simulink model "EspacioEstado"  (R2017b)
settings: Solver=VariableStepAuto  StartTime=0.0  StopTime=0.5  MaxStep=1e-4  RelTol=1e-3
values from neighbouring files (symbols this model uses):
  A = pi()*((D/2)^2)    [MODELOHIDRO.m]    (also in MODELOHIDROV10.m; MODELOHIDROV2.m; MODELOHIDROV3.m; MODELOHIDROV4.m)
  B = 0    [MODELOHIDRO.m]    (also in MODELOHIDROV10.m; MODELOHIDROV2.m; MODELOHIDROV3.m; MODELOHIDROV4.m)
  C = [1 0;0 1]    [PruebaDCDC.m]    (also in stateStadeInv.m = [0 0 0 1 0 0;0 0 0 0 1 0;0 0 0 0 0 1])
  Ccc = 2.5e-3    (= 0.0025)    [MODELOHIDROV4.m]    (also in MODELOHIDROV7.m = 8.33e-05; MODELOHIDROV8.m = 8.33e-05; PruebaDCDC.m = 8.33e-05)
  D = 1    [MODELOHIDRO.m]    (also in MODELOHIDROV10.m; MODELOHIDROV2.m; MODELOHIDROV3.m; MODELOHIDROV4.m)
  Dcc = 0.625    [MODELOHIDROV4.m]    (also in MODELOHIDROV7.m; MODELOHIDROV8.m; PruebaDCDC.m)
  Lcc = 70.3e-6    (= 7.03e-05)    [MODELOHIDROV4.m]    (also in MODELOHIDROV7.m = 0.002109; MODELOHIDROV8.m = 0.002109; PruebaDCDC.m = 0.002109)
  Rcc = 7.5    [MODELOHIDROV4.m]    (also in MODELOHIDROV7.m = 225; MODELOHIDROV8.m = 225; PruebaDCDC.m = 225)
libraries: powerlib x1
settings Model: Creator=Hp 14  LastModifiedBy=Hp 14

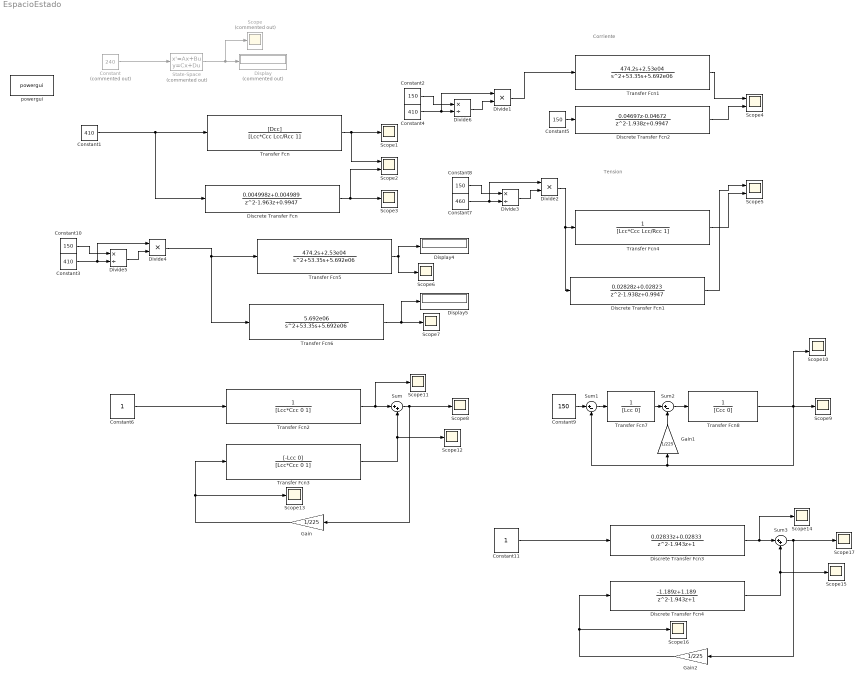
== system EspacioEstado ==
  note: Tension
  note: Corriente
  Constant : Constant  Commented=on  Value=240
  Constant1 : Constant  Value=410
  Constant{2,5,8..10} (5 alike) : Constant  Value=150
  Constant11 : Constant
  Constant3 : Constant  Value=410
  Constant4 : Constant  Value=410
  Constant6 : Constant
  Constant7 : Constant  Value=460
  Discrete Transfer Fcn : DiscreteTransferFcn  Numerator=[0.004998 0.004989]  Denominator=[1 -1.963 0.9947]
  Discrete Transfer Fcn1 : DiscreteTransferFcn  Numerator=[0.02828 0.02823]  Denominator=[1 -1.938 0.9947]
  Discrete Transfer Fcn2 : DiscreteTransferFcn  Numerator=[0.04697 -0.04672]  Denominator=[1 -1.938 0.9947]
  Discrete Transfer Fcn3 : DiscreteTransferFcn  Numerator=[0.02833 0.02833]  Denominator=[1 -1.943 1]
  Discrete Transfer Fcn4 : DiscreteTransferFcn  Numerator=[-1.189 1.189]  Denominator=[1 -1.943 1]
  Display : Display  Commented=on
  Display4 : Display
  Display5 : Display
  Divide1 : Product  Inputs=**
  Divide2 : Product  Inputs=**
  Divide3 : Product  Inputs=*/
  Divide4 : Product  Inputs=**
  Divide5 : Product  Inputs=*/
  Divide6 : Product  Inputs=*/
  Gain : Gain  Gain=1/225
  Gain1 : Gain  Gain=1/225
  Gain2 : Gain  Gain=1/225
  Scope : Scope  Commented=on
  Scope{1,3,6..9,11..17} (13 alike) : Scope
  Scope{2,4..5,10} (4 alike) : Scope  NumInputPorts=2
  State-Space : StateSpace  Commented=on  A=A  B=B  C=C  D=D  InitialCondition=0
  Sum : Sum  Inputs=|++
  Sum1 : Sum  Inputs=|+-
  Sum2 : Sum  Inputs=|+-
  Sum3 : Sum  Inputs=|++
  Transfer Fcn : TransferFcn  Numerator=[Dcc]  Denominator=[Lcc*Ccc Lcc/Rcc 1]
  Transfer Fcn1 : TransferFcn  Numerator=[474.2 2.53e04]  Denominator=[1 53.35 5.692e06]
  Transfer Fcn2 : TransferFcn  Denominator=[Lcc*Ccc 0 1]
  Transfer Fcn3 : TransferFcn  Numerator=[-Lcc 0]  Denominator=[Lcc*Ccc 0 1]
  Transfer Fcn4 : TransferFcn  Denominator=[Lcc*Ccc Lcc/Rcc 1]
  Transfer Fcn5 : TransferFcn  Numerator=[474.2 2.53e04]  Denominator=[1 53.35 5.692e06]
  Transfer Fcn6 : TransferFcn  Numerator=[5.692e06]  Denominator=[1 53.35 5.692e06]
  Transfer Fcn7 : TransferFcn  Denominator=[Lcc 0]
  Transfer Fcn8 : TransferFcn  Denominator=[Ccc 0]
  powergui : powerlib/powergui  Priority=1  SimulationMode=Continuous  SampleTime=50e-3  frequency=60  Iterations=50  frequencyindice=0  Pbase=100e6  ErrMax=1e-4  UnitsV=kV  UnitsW=MW  buscounter=0  FunctionMessages=off  echomessages=off  EnableUseOfTLC=off  CurrentSourceSwitches=off  DisableSnubberDevices=off  DisableRonSwitches=off  DisableVfSwitches=off  DisplayEquations=off  SolverType=Tustin/Backward Euler (TBE)  Interpol=off  ExternalGateDelay=off  methode=off  Ts=100  x0status=blocks  SPID=on  SwTol=0  HookPort=off  RestoreLinks=warning  ResistiveCurrentMeasurement=off  Frange=[0:2:500]  Ylog=off  Xlog=on  ShowGrid=off  save=off  variable=ZData  structure=0  ZoomFFT=off  StartTime=0.0  cycles=1  DisplayStyle=1  fundamental=60  FreqAxis=off  MaxFrequency=1000  frequencyindicesteady=0 Hz  RmsSteady=1  display=off
  wires:
  Constant/1 -> State-Space/1
  State-Space/1 -> Scope/1, Display/1
  Transfer Fcn/1 -> Scope2/1, Scope1/1
  Constant1/1 -> Discrete Transfer Fcn/1, Transfer Fcn/1
  Discrete Transfer Fcn/1 -> Scope3/1, Scope2/2
  Constant7/1 -> Divide3/2, Divide2/1
  Constant8/1 -> Divide3/1
  Divide3/1 -> Divide2/2
  Divide2/1 -> Transfer Fcn4/1, Discrete Transfer Fcn1/1
  Discrete Transfer Fcn1/1 -> Scope5/1
  Transfer Fcn4/1 -> Scope5/2
  Transfer Fcn5/1 -> Display4/1, Scope6/1
  Transfer Fcn6/1 -> Display5/1, Scope7/1
  Divide5/1 -> Divide4/2
  Constant10/1 -> Divide5/1
  Constant3/1 -> Divide4/1, Divide5/2
  Divide4/1 -> Transfer Fcn6/1, Transfer Fcn5/1
  Divide1/1 -> Transfer Fcn1/1
  Constant4/1 -> Divide6/2, Divide1/1
  Constant2/1 -> Divide6/1
  Divide6/1 -> Divide1/2
  Transfer Fcn1/1 -> Scope4/1
  Discrete Transfer Fcn2/1 -> Scope4/2
  Constant5/1 -> Discrete Transfer Fcn2/1
  Transfer Fcn2/1 -> Scope11/1, Sum/1
  Transfer Fcn3/1 -> Scope12/1, Sum/2
  Sum/1 -> Scope8/1, Gain/1
  Gain/1 -> Scope13/1, Transfer Fcn3/1
  Constant6/1 -> Transfer Fcn2/1
  Constant9/1 -> Sum1/1
  Sum1/1 -> Transfer Fcn7/1
  Transfer Fcn7/1 -> Sum2/1
  Sum2/1 -> Transfer Fcn8/1
  Transfer Fcn8/1 -> Sum1/2, Gain1/1, Scope10/2, Scope9/1
  Gain1/1 -> Sum2/2
  Constant11/1 -> Discrete Transfer Fcn3/1
  Gain2/1 -> Discrete Transfer Fcn4/1, Scope16/1
  Sum3/1 -> Gain2/1, Scope17/1
  Discrete Transfer Fcn4/1 -> Sum3/2, Scope15/1
  Discrete Transfer Fcn3/1 -> Sum3/1, Scope14/1
